simulink model "invPendPid2"  (R2022a)
settings: Solver=VariableStepAuto  StartTime=0.0  StopTime=10.0  RelTol=1e-3
settings Model: Creator=Shiva  LastModifiedBy=Shiva

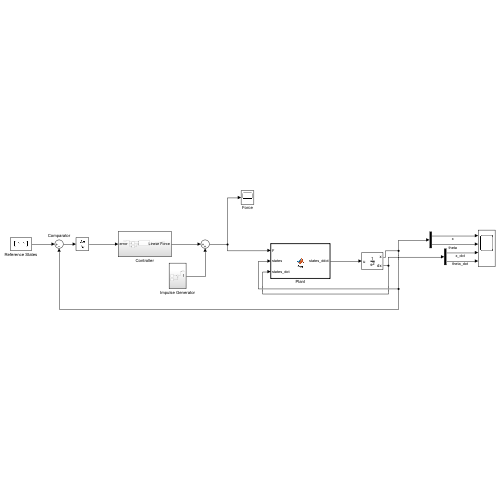
[thumbnail: Simulink's stored preview of the top-level diagram]
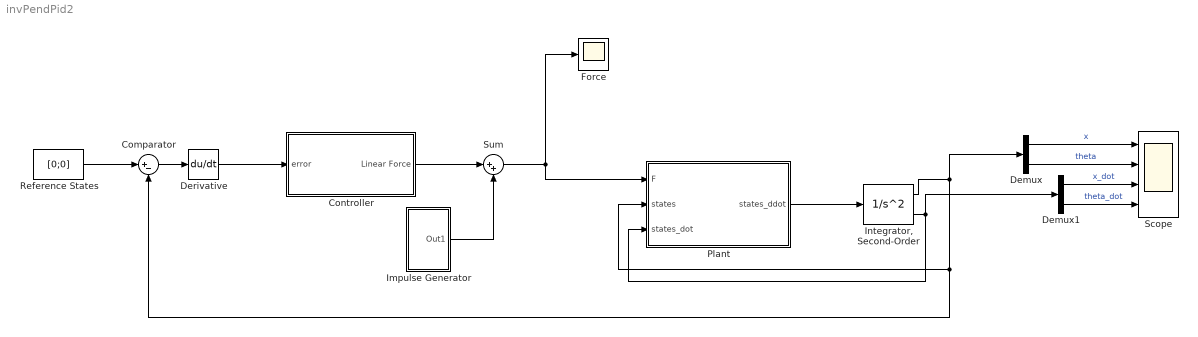
== system invPendPid2 ==
  Comparator : Sum  Inputs=|+-
  Controller : Subsystem
  Demux : Demux  Outputs=2
  Demux1 : Demux  Outputs=2
  Derivative : Derivative
  Force : Scope
  Impulse Generator : Subsystem
  "Integrator, Second-Order" : SecondOrderIntegrator  ICX=[0,0]  ICDXDT=[0,0]
  Plant : MATLAB Function  TreatAsAtomicUnit=on
  Reference States : Constant  Value=[0;0]  SampleTime=1
  Scope : Scope  NumInputPorts=4
  Sum : Sum  Inputs=|++
  wires:
  Plant/1(states_ddot) -> "Integrator, Second-Order"/1
  "Integrator, Second-Order"/1 -> Comparator/2, Plant/2(states), Demux/1
  "Integrator, Second-Order"/2 -> Demux1/1, Plant/3(states_dot)
  Reference States/1 -> Comparator/1
  Demux/1 -> Scope/1  "x"
  Demux/2 -> Scope/2  "theta"
  Demux1/1 -> Scope/3  "x_dot"
  Demux1/2 -> Scope/4  "theta_dot"
  Sum/1 -> Plant/1(F), Force/1
  Controller/1(Linear Force) -> Sum/1
  Impulse Generator/1(Out1) -> Sum/2
  Comparator/1 -> Derivative/1
  Derivative/1 -> Controller/1(error)

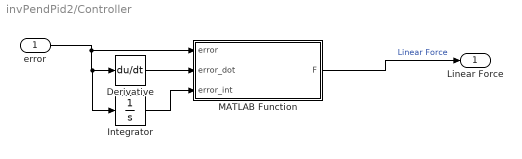
== system invPendPid2/Controller ==
  error : Inport
  Derivative : Derivative
  Integrator : Integrator
  MATLAB Function : MATLAB Function  TreatAsAtomicUnit=on
  Linear Force : Outport
  wires:
  error/1 -> Integrator/1, Derivative/1, MATLAB Function/1(error)
  MATLAB Function/1(F) -> Linear Force/1  "Linear Force"
  Derivative/1 -> MATLAB Function/2(error_dot)
  Integrator/1 -> MATLAB Function/3(error_int)

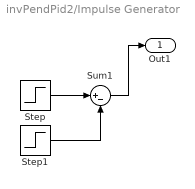
== system invPendPid2/Impulse Generator ==
  Step : Step  After=0.1  SampleTime=1
  Step1 : Step  Time=2  After=0.1  SampleTime=1
  Sum1 : Sum  Inputs=|+-
  Out1 : Outport
  wires:
  Step1/1 -> Sum1/2
  Step/1 -> Sum1/1
  Sum1/1 -> Out1/1

== matlab function invPendPid2/Controller/MATLAB Function ==
  data: error input; F output; error_dot input; error_int input
function F = fcn(error,error_dot,error_int)

M1=0.121;
M2=0.086;
L=0.3;
g=9.81;

Kp=10;
Kd=1;
Ki=1;

error_ddot=-Kp.*error(1)-Kd.*error_dot(1)-Ki*error_int(1);

F=-error_ddot*(M1+M2*(1-0.75*cos(error(2))*cos(error(2))))-0.75*M2*g*sin(error(2))*cos(error(2))+0.5*M2*L*error_dot(2)*error_dot(2)*sin(error(2));

% states_ddot=[(F+0.75*M2*g*sin(states(2))*cos(states(2))-0.5*M2*L*states_dot(2)*states_dot(2)*sin(states(2)))/(M1+M2*(1-0.75*cos(states(2))*cos(states(2))));
%     1.5*((M1+M2)*g*sin(states(2))+F*cos(states(2))-0.5*M2*L*states_dot(2)*states_dot(2)*sin(states(2))*cos(states(2)))/(L*(M1+M2*(1-0.75*cos(states(2))*cos(states(2)))))];

== matlab function invPendPid2/Plant ==
  data: F input; states_ddot output; states input; states_dot input
function states_ddot = fcn(F,states, states_dot)
M1=0.121;
M2=0.086;
L=0.3;
g=9.81;
states_ddot=[(F+0.75*M2*g*sin(states(2))*cos(states(2))-0.5*M2*L*states_dot(2)*states_dot(2)*sin(states(2)))/(M1+M2*(1-0.75*cos(states(2))*cos(states(2))));
    1.5*((M1+M2)*g*sin(states(2))+F*cos(states(2))-0.5*M2*L*states_dot(2)*states_dot(2)*sin(states(2))*cos(states(2)))/(L*(M1+M2*(1-0.75*cos(states(2))*cos(states(2)))))];
